simulink subsystem "Controller"  (R2022a)
settings: Solver=VariableStepAuto  StartTime=0.0  StopTime=10.0  RelTol=1e-3
libraries: simulink x3
settings Model: Creator=Haier  LastModifiedBy=Haier

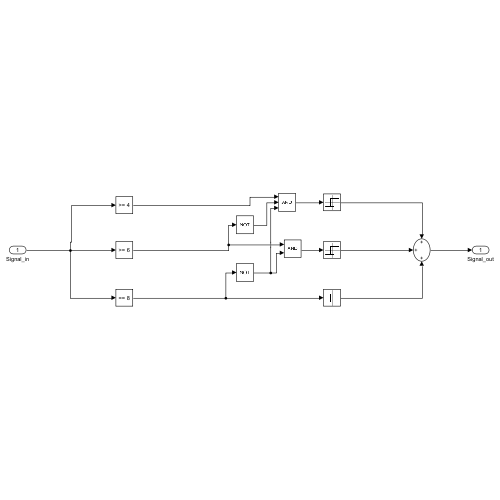
[thumbnail: Simulink's stored preview of the top-level diagram]
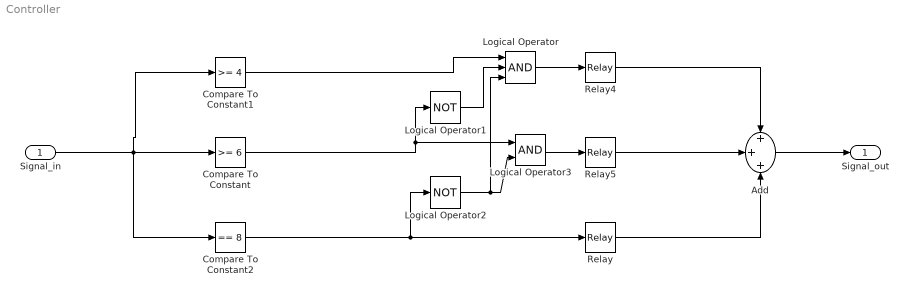
== system Controller ==
  Signal_in : Inport
  Add : Sum  Inputs=+++
  Compare To Constant : simulink/Logic and Bit Operations/Compare To Constant  relop=>=  const=6  OutDataTypeStr=boolean
  Compare To Constant1 : simulink/Logic and Bit Operations/Compare To Constant  relop=>=  const=4  OutDataTypeStr=boolean
  Compare To Constant2 : simulink/Logic and Bit Operations/Compare To Constant  relop===  const=8  OutDataTypeStr=boolean
  Logical Operator : Logic  Inputs=3  AllPortsSameDT=off  OutDataTypeStr=boolean
  Logical Operator1 : Logic  Operator=NOT  AllPortsSameDT=off  OutDataTypeStr=boolean
  Logical Operator2 : Logic  Operator=NOT  AllPortsSameDT=off  OutDataTypeStr=boolean
  Logical Operator3 : Logic  AllPortsSameDT=off  OutDataTypeStr=boolean
  Relay : Relay  OnSwitchValue=1  OffSwitchValue=0  OnOutputValue=4  OutDataTypeStr=double
  Relay4 : Relay  OnSwitchValue=1  OffSwitchValue=0  OnOutputValue=2  OutDataTypeStr=double
  Relay5 : Relay  OnSwitchValue=1  OffSwitchValue=0  OnOutputValue=3  OutDataTypeStr=double
  Signal_out : Outport
  wires:
  Relay/1 -> Add/3
  Signal_in/1 -> Compare To Constant/1, Compare To Constant2/1, Compare To Constant1/1
  Logical Operator3/1 -> Relay5/1
  Logical Operator2/1 -> Logical Operator/3, Logical Operator3/2
  Logical Operator/1 -> Relay4/1
  Logical Operator1/1 -> Logical Operator/2
  Compare To Constant/1 -> Logical Operator1/1, Logical Operator3/1
  Compare To Constant1/1 -> Logical Operator/1
  Compare To Constant2/1 -> Logical Operator2/1, Relay/1
  Relay4/1 -> Add/1
  Add/1 -> Signal_out/1
  Relay5/1 -> Add/2
